simulink model "Capstone_SimV2_Fluid_Tube_Added"  (R2023b)
settings: Solver=VariableStepAuto  StartTime=0.0  StopTime=10  FixedStep=0.001  RelTol=1e-3
values from neighbouring files (symbols this model uses):
  A_membrane = 0.01    [Capstone_Model.m]    (also in Capstone_Model_V2.m)
  A_tube = pi*(D_tube/2)^2    (= 3.16692174436e-05)    [Capstone_Model_V2.m]
  bpm = 80    [Capstone_Model_V2.m]
  C_membrane = 100    [Capstone_Model.m]    (also in Capstone_Model_V2.m)
  D_tube = 0.00635    [Capstone_Model_V2.m]
  duty_cycle = 0.4    [Capstone_Model_V2.m]
  K_membrane = 1000    [Capstone_Model_V2.m]
  L_membrane = 0.9144    [Capstone_Model_V2.m]
  L_stopcock = 0.9144    [Capstone_Model_V2.m]
  mu = 0.001    [Capstone_Model_V2.m]
  P_reservoir = 0    [Capstone_Model_V2.m]
  Q_pump_max = 0.000133    [Capstone_Model_V2.m]
  rho = 1000    [Capstone_Model_V2.m]
  V0 = 0.01    [Capstone_Model.m]    (also in Capstone_Model_V2.m = 0.0005)
settings Model: Creator=johny  LastModifiedBy=johny

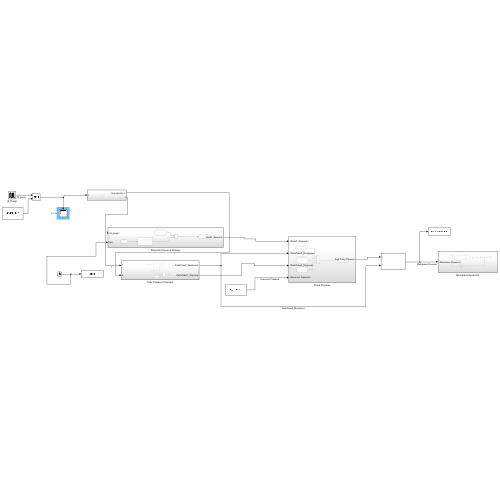
[thumbnail: Simulink's stored preview of the top-level diagram]
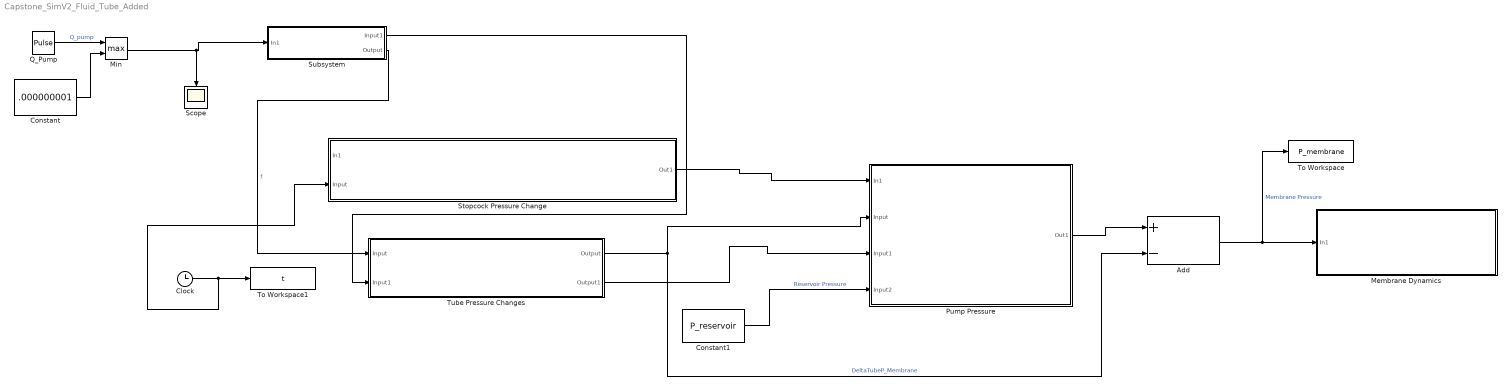
== system Capstone_SimV2_Fluid_Tube_Added ==
  Add : Sum  Inputs=+-
  Clock : Clock
  Constant : Constant  Value=.000000001
  Constant1 : Constant  Value=P_reservoir
  Membrane Dynamics : Subsystem
  Min : MinMax  Function=max  Inputs=2
  Pump Pressure : Subsystem
  Q_Pump : DiscretePulseGenerator  PulseType=Time based  Amplitude=Q_pump_max  Period=60/bpm  PulseWidth=duty_cycle*100
  Scope : Scope
  Stopcock Pressure Change : Subsystem
  Subsystem : Subsystem
  To Workspace : ToWorkspace  VariableName=P_membrane  SampleTime=-1
  To Workspace1 : ToWorkspace  VariableName=t  SampleTime=-1
  Tube Pressure Changes : Subsystem
  wires:
  Stopcock Pressure Change/1(Out1) -> Pump Pressure/1(In1)
  Tube Pressure Changes/2(Output1) -> Pump Pressure/3(Input1)
  Tube Pressure Changes/1(Output) -> Add/2, Pump Pressure/2(Input)  "DeltaTubeP_Membrane"
  Constant1/1 -> Pump Pressure/4(Input2)  "Reservoir Pressure"
  Pump Pressure/1(Out1) -> Add/1
  Add/1 -> To Workspace/1, Membrane Dynamics/1(In1)  "Membrane Pressure"
  Clock/1 -> Stopcock Pressure Change/2(Input), To Workspace1/1
  Subsystem/2(Output) -> Tube Pressure Changes/1(Input)  "f"
  Subsystem/1(Input1) -> Tube Pressure Changes/2(Input1)
  Constant/1 -> Min/2
  Q_Pump/1 -> Min/1  "Q_pump"
  Min/1 -> Scope/1, Subsystem/1(In1)

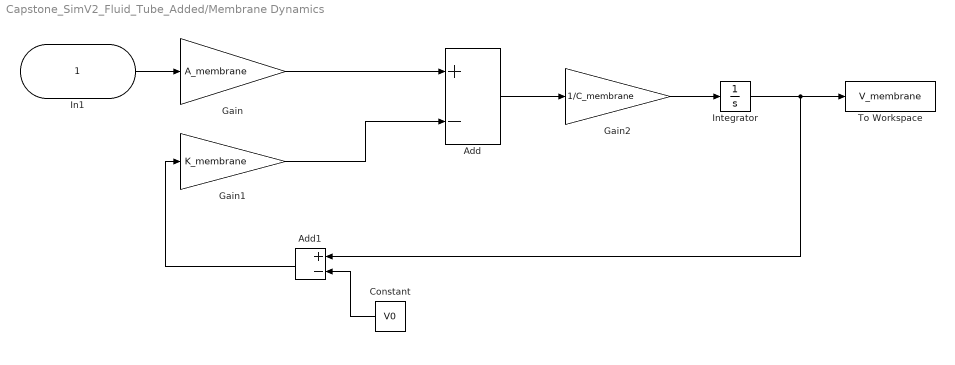
== system Capstone_SimV2_Fluid_Tube_Added/Membrane Dynamics ==
  In1 : Inport
  Add : Sum  Inputs=+-
  Add1 : Sum  Inputs=+-
  Constant : Constant  Value=V0
  Gain : Gain  Gain=A_membrane
  Gain1 : Gain  Gain=K_membrane
  Gain2 : Gain  Gain=1/C_membrane
  Integrator : Integrator  InitialCondition=V0
  To Workspace : ToWorkspace  VariableName=V_membrane  SampleTime=-1
  wires:
  In1/1 -> Gain/1
  Gain/1 -> Add/1
  Gain1/1 -> Add/2
  Constant/1 -> Add1/2
  Add1/1 -> Gain1/1
  Add/1 -> Gain2/1
  Integrator/1 -> Add1/1, To Workspace/1
  Gain2/1 -> Integrator/1

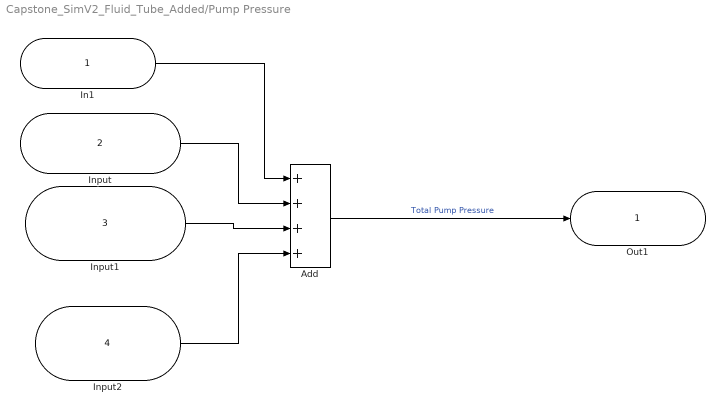
== system Capstone_SimV2_Fluid_Tube_Added/Pump Pressure ==
  In1 : Inport
  Input : Inport  Port=2
  Input1 : Inport  Port=3
  Input2 : Inport  Port=4
  Add : Sum  Inputs=++++
  Out1 : Outport
  wires:
  Input2/1 -> Add/4
  Input1/1 -> Add/3
  Input/1 -> Add/2
  In1/1 -> Add/1
  Add/1 -> Out1/1  "Total Pump Pressure"

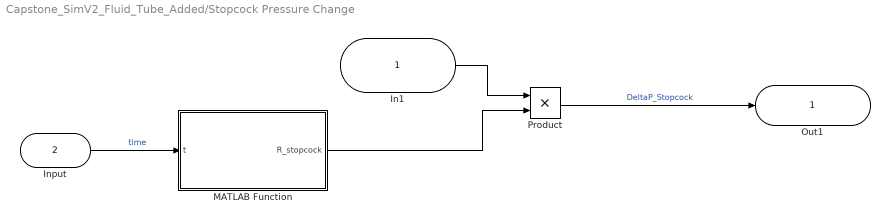
== system Capstone_SimV2_Fluid_Tube_Added/Stopcock Pressure Change ==
  In1 : Inport
  Input : Inport  Port=2
  MATLAB Function : MATLAB Function  TreatAsAtomicUnit=on
  Product : Product
  Out1 : Outport
  wires:
  MATLAB Function/1(R_stopcock) -> Product/2
  In1/1 -> Product/1
  Product/1 -> Out1/1  "DeltaP_Stopcock"
  Input/1 -> MATLAB Function/1(t)  "time"

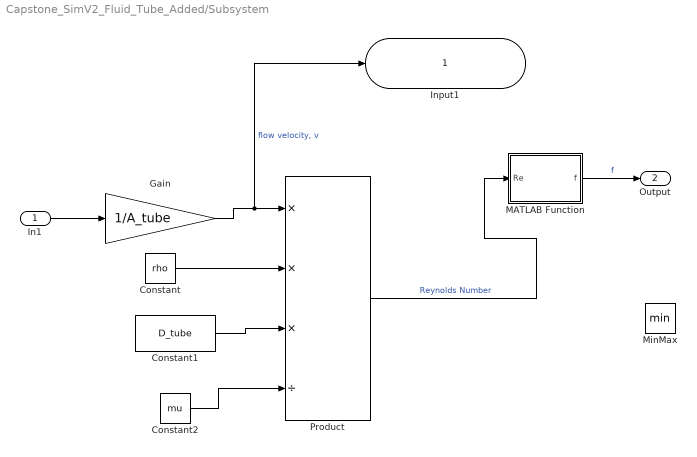
== system Capstone_SimV2_Fluid_Tube_Added/Subsystem ==
  In1 : Inport
  Constant : Constant  Value=rho
  Constant1 : Constant  Value=D_tube
  Constant2 : Constant  Value=mu
  Gain : Gain  Gain=1/A_tube
  MATLAB Function : MATLAB Function  TreatAsAtomicUnit=on
  MinMax : MinMax
  Product : Product  Inputs=***/
  Input1 : Outport
  Output : Outport  Port=2
  wires:
  In1/1 -> Gain/1
  Gain/1 -> Input1/1, Product/1  "flow velocity, v"
  Product/1 -> MATLAB Function/1(Re)  "Reynolds Number"
  Constant/1 -> Product/2
  Constant1/1 -> Product/3
  Constant2/1 -> Product/4
  MATLAB Function/1(f) -> Output/1  "f"

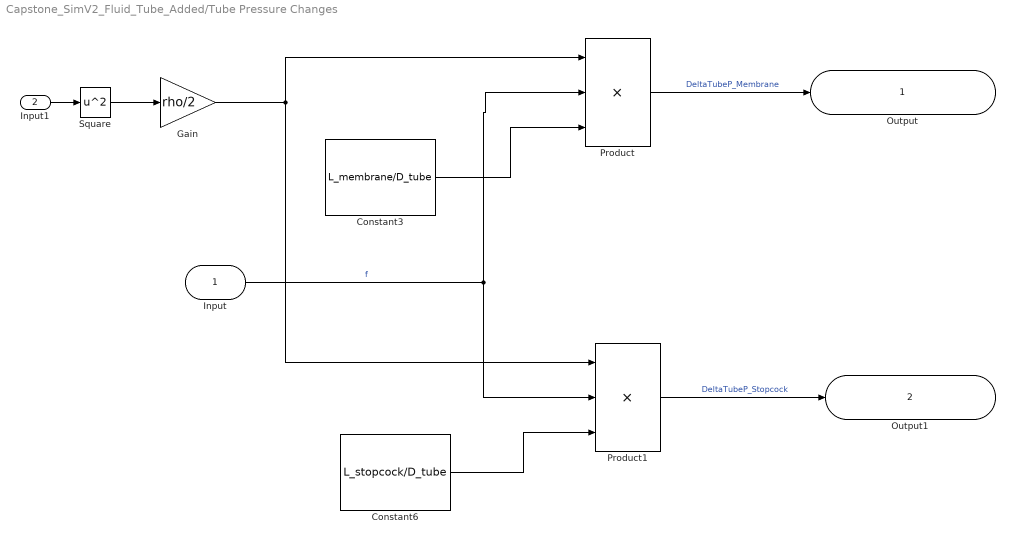
== system Capstone_SimV2_Fluid_Tube_Added/Tube Pressure Changes ==
  Input : Inport
  Input1 : Inport  Port=2
  Constant3 : Constant  Value=L_membrane/D_tube
  Constant6 : Constant  Value=L_stopcock/D_tube
  Gain : Gain  Gain=rho/2
  Product : Product  Inputs=3
  Product1 : Product  Inputs=3
  Square : Math  Operator=square
  Output : Outport
  Output1 : Outport  Port=2
  wires:
  Constant3/1 -> Product/3
  Constant6/1 -> Product1/3
  Product1/1 -> Output1/1  "DeltaTubeP_Stopcock"
  Product/1 -> Output/1  "DeltaTubeP_Membrane"
  Input/1 -> Product/2, Product1/2  "f"
  Input1/1 -> Square/1
  Square/1 -> Gain/1
  Gain/1 -> Product/1, Product1/1

== matlab function Capstone_SimV2_Fluid_Tube_Added/Stopcock Pressure Change/MATLAB Function ==
  data: t input; R_stopcock output
function R_stopcock = dynamicResistance(t)
    R_base = 1e5; % Base resistance [Pa·s/m^3]
    R_amplitude = 4e5; % Amplitude of resistance variation
    freq = 1; % Frequency of oscillation [Hz]
    R_stopcock = R_base+R_amplitude*sin(2*pi*freq*t);
end

== matlab function Capstone_SimV2_Fluid_Tube_Added/Subsystem/MATLAB Function ==
  data: Re input; f output
function f = friction_factor(Re)
    if Re < 2300
        f = 64 / Re; % Laminar flow
    else
        f = 0.3164 / (Re^(1/4)); % Turbulent flow
    end
end
